simulink model "Inc_conductance"  (R2014a)
settings: Solver=ode45  StartTime=0.0  StopTime=10.0  RelTol=1e-3
settings Model: Creator=kartik.karuna  LastModifiedBy=kartik.karuna

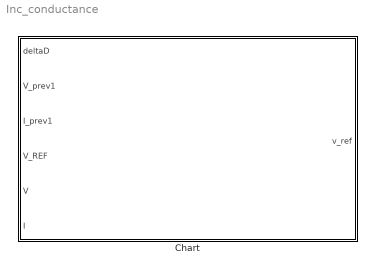
== system Inc_conductance ==
  Chart : Stateflow chart  TreatAsAtomicUnit=on

== stateflow chart Inc_conductance/Chart ==
  state Sample_and_call
    entry:
    deltaV = V -V_prev1;
    deltaI = I - I_prev1;
    v_ref = V_REF;
  state INCREMENT
    entry:
    v_ref =v_ref+deltaD;
  state DECREMENT
    entry:
    v_ref =v_ref-deltaD;
  state RETURN
    entry:
    V_prev1 = V;
    I_prev1 = I ;
    V_REF= v_ref;
  (default) -> Sample_and_call
  RETURN -> Sample_and_call
  Sample_and_call -> (junction 6) [order 1] : [deltaV==0]
  Sample_and_call -> (junction 22) [order 2] : [deltaV~=0]
  (junction 6) -> RETURN [order 2] : [deltaI==0]
  (junction 6) -> (junction 16) [order 1] : [deltaI~=0]
  (junction 22) -> RETURN [order 2] : [deltaI/deltaV == -(I/V)]
  (junction 22) -> (junction 15) [order 1] : [deltaI/deltaV ~= -(I/V)]
  (junction 16) -> DECREMENT [order 2] : [deltaI<=0]
  (junction 16) -> INCREMENT [order 1] : [deltaI>0]
  (junction 15) -> INCREMENT [order 1] : [deltaI/deltaV > -(I/V)]
  (junction 15) -> DECREMENT [order 2] : [deltaI/deltaV <= -(I/V)]
  INCREMENT -> RETURN
  DECREMENT -> RETURN
  data: deltaD input; v_ref output; V_prev1 input; I_prev1 input; V_REF input; deltaV local; deltaI local; V input; I input
